simulink model "dynamiczny_ciagly_dyskretny"  (R2020a)
settings: Solver=VariableStepAuto  StartTime=0.0  StopTime=100  RelTol=1e-3
values from neighbouring files (symbols this model uses):
  a1 = 0.56    [init_values.m]
  a2 = -0.8    [init_values.m]
  a3 = -0.25    [init_values.m]
  a4 = 0.2    [init_values.m]
  K = 4    [init_values.m]
  T = 1    [test.m]    (also in zad1_10.m; zad1_3.m = 0.1; zad1_9.m)
  T1 = 4    [init_values.m]
  T2 = 10    [init_values.m]
settings Model: Creator=jakub  LastModifiedBy=jakub

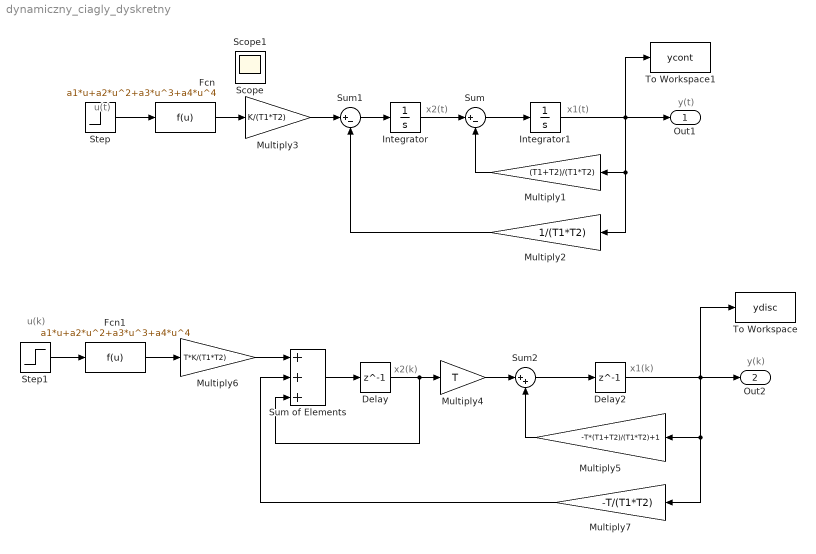
== system dynamiczny_ciagly_dyskretny ==
  note: u(t)
  note: y(t)
  note: x1(t)
  note: x2(t)
  note: u(k)
  note: x1(k)
  note: y(k)
  note: x2(k)
  Delay : Delay  DelayLength=1  InitialCondition=0  SampleTime=T
  Delay2 : Delay  DelayLength=1  InitialCondition=0  SampleTime=T
  Fcn : Fcn  Expr=a1*u+a2*u^2+a3*u^3+a4*u^4
  Fcn1 : Fcn  Expr=a1*u+a2*u^2+a3*u^3+a4*u^4
  Integrator : Integrator  ZeroCross=off
  Integrator1 : Integrator  ZeroCross=off
  Multiply1 : Gain  Gain=(T1+T2)/(T1*T2)
  Multiply2 : Gain  Gain=1/(T1*T2)
  Multiply3 : Gain  Gain=K/(T1*T2)
  Multiply4 : Gain  Gain=T
  Multiply5 : Gain  Gain=-T*(T1+T2)/(T1*T2)+1
  Multiply6 : Gain  Gain=T*K/(T1*T2)
  Multiply7 : Gain  Gain=-T/(T1*T2)
  Step : Step  SampleTime=0
  Step1 : Step  SampleTime=0
  Sum : Sum  Inputs=|+-
  Sum of Elements : Sum  Inputs=+++
  Sum1 : Sum  Inputs=|+-
  Sum2 : Sum  Inputs=|++
  To Workspace : ToWorkspace  VariableName=ydisc  SaveFormat=Structure With Time  SampleTime=T
  To Workspace1 : ToWorkspace  VariableName=ycont  SaveFormat=Structure With Time  SampleTime=-1
  Out1 : Outport
  Out2 : Outport  Port=2
  Scope : Scope
  Scope1 : Scope
  wires:
  Integrator1/1 -> Multiply2/1, Multiply1/1, Out1/1, To Workspace1/1
  Multiply1/1 -> Sum/2
  Integrator/1 -> Sum/1
  Sum/1 -> Integrator1/1
  Multiply2/1 -> Sum1/2
  Sum1/1 -> Integrator/1
  Multiply3/1 -> Sum1/1
  Step/1 -> Fcn/1
  Fcn/1 -> Multiply3/1
  Multiply7/1 -> Sum of Elements/2
  Multiply4/1 -> Sum2/1
  Multiply6/1 -> Sum of Elements/1
  Delay2/1 -> To Workspace/1, Out2/1, Multiply5/1, Multiply7/1
  Fcn1/1 -> Multiply6/1
  Multiply5/1 -> Sum2/2
  Sum of Elements/1 -> Delay/1
  Delay/1 -> Sum of Elements/3, Multiply4/1
  Step1/1 -> Fcn1/1
  Sum2/1 -> Delay2/1
